simulink model "plant"  (R2022a)
settings: Solver=FixedStepAuto  StartTime=0.0  StopTime=Inf  FixedStep=Ts  RelTol=1e-3  EnableMultiTasking=on
undefined symbols (not defined in the file): A, Analog_max, Calib_Gain, Cd, Crr, D, DiscIntNeverNeededParam, eff_gear, g, Ipeak, Ke, Kf, Kt, La, m_total, n_gear, Offset, Ra, rho, Rwheel, Ts, V_AImax, Vbat, w_motor_max
libraries: c2837xDlib x4, c280xlib x2, simulink x1, c2802xlib x1
settings Model: ExtModeTrigDuration=8  Creator=34688  LastModifiedBy=manu.sanchez
settings SolverCC: AutoInsertRateTranBlk=on
settings OptimizationCC: DefaultUnderspecifiedDataType=single  EnhancedBackFolding=on  PassReuseOutputArgsAs=Individual arguments  MaxStackSize=1024  OptimizeBlockOrder=speed  DifferentSizesBufferReuse=on  OptimizationCustomize=off  DenormalBehavior=FlushToZero  EfficientTunableParamExpr=on
settings DebuggingCC: ParameterTunabilityLossMsg=error  UnconnectedInputMsg=warning  UnconnectedOutputMsg=warning  UnconnectedLineMsg=warning
settings HardwareCC: ProdBitPerChar=16  ProdBitPerInt=16  ProdBitPerPointer=32  ProdBitPerSizeT=32  ProdBitPerPtrDiffT=32  ProdLargestAtomicInteger=Integer  ProdLargestAtomicFloat=None  ProdWordSize=16  ProdLongLongMode=on  ProdHWDeviceType=Texas Instruments->C2000
settings SFSimCC: MATLABDynamicMemAlloc=off
settings RTWCC: SystemTargetFile=ert.tlc  HardwareBoard=TI Delfino F28379D LaunchPad  TemplateMakefile=ert_default_tmf  Toolchain=Texas Instruments Code Composer Studio (C2000)  DLArmComputeVersion=19.05
settings CodeAppCC: ForceParamTrailComments=on  IgnoreCustomStorageClasses=off  OperatorAnnotations=on  SimulinkDataObjDesc=on  SFDataObjDesc=on  InsertBlockDesc=on
settings ERTTargetCC: CodeReplacementLibrary=TI C28x  SupportContinuousTime=on  ExtModeTransport=3  ExtModeStaticAllocSize=10000

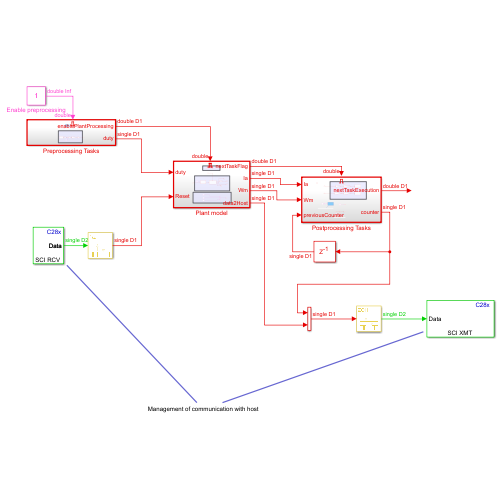
[thumbnail: Simulink's stored preview of the top-level diagram]
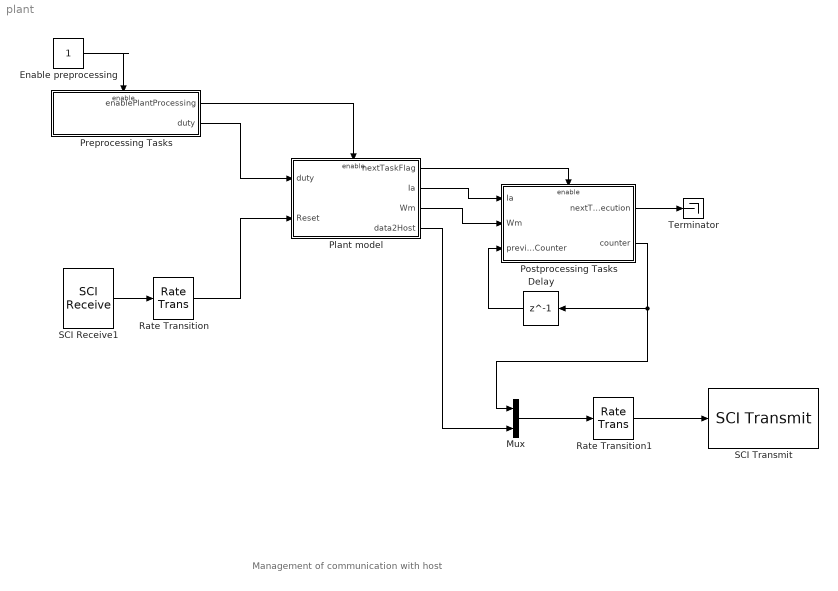
== system plant ==
  note: Management of communication with host
  Delay : Delay  DelayLength=1
  Enable preprocessing : Constant
  Mux : Mux  Inputs=2
  Plant model : Subsystem  TreatAsAtomicUnit=on
  Postprocessing Tasks : Subsystem  TreatAsAtomicUnit=on
  Preprocessing Tasks : Subsystem  TreatAsAtomicUnit=on
  Rate Transition : RateTransition  OutPortSampleTime=Ts
  Rate Transition1 : RateTransition  OutPortSampleTime=1e-3
  SCI Receive1 : c280xlib/SCI Receive  sciModule=A  dataHead='S'  headerCheckMaxCount=16  dataTail='E'  dataType=single  dataLenOptions=Length via dialog  dataDim=1  maxDataLength=1  initValue=0  errOption=Output the last received value  errValue=0  sampleTime=0.001  blockingMode=on  timeOut=0.00875  outputStatus=off
      settings: SourceProductBaseCode=TIC2000
  SCI Transmit : c280xlib/SCI Transmit  sciModule=A  dataHead='S'  dataTail='E'  blockingMode=on  outputStatus=off
  Terminator : Terminator
  wires:
  Plant model/1(nextTaskFlag) -> Postprocessing Tasks/Enable
  Plant model/2(Ia) -> Postprocessing Tasks/1(Ia)
  Enable preprocessing/1 -> Preprocessing Tasks/Enable
  Preprocessing Tasks/1(enablePlantProcessing) -> Plant model/Enable
  Rate Transition/1 -> Plant model/2(Reset)
  SCI Receive1/1 -> Rate Transition/1
  Rate Transition1/1 -> SCI Transmit/1
  Postprocessing Tasks/1(nextTaskExecution) -> Terminator/1
  Delay/1 -> Postprocessing Tasks/3(previousCounter)
  Postprocessing Tasks/2(counter) -> Mux/1, Delay/1
  Mux/1 -> Rate Transition1/1
  Plant model/4(data2Host) -> Mux/2
  Preprocessing Tasks/2(duty) -> Plant model/1(duty)
  Plant model/3(Wm) -> Postprocessing Tasks/2(Wm)

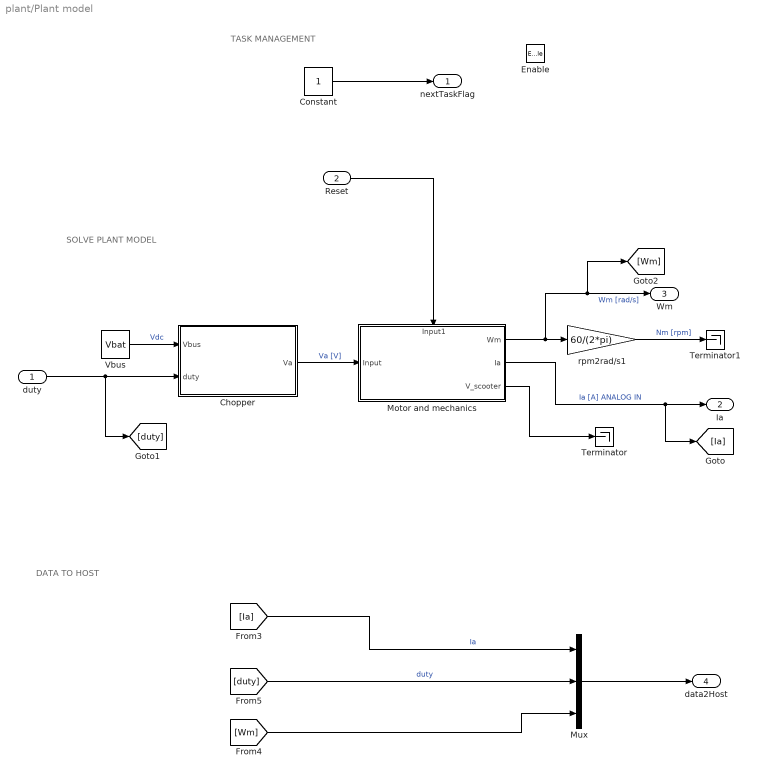
== system plant/Plant model ==
  note: TASK MANAGEMENT
  note: SOLVE PLANT MODEL
  note: DATA TO HOST
  duty : Inport
  Reset : Inport  Port=2
  Enable : EnablePort
  Chopper : Subsystem  Variant=on  VariantControlMode=label  LabelModeActiveChoice=HALF_BRIDGE  mask{LabelModeActiveChoice=HALF_BRIDGE}
      mask prompts: LabelModeActiveChoice "Simulink:Variants:LabelComboBox"
      mask TypeOptions LabelModeActiveChoice: LabelModeActiveChoice
      mask DialogControl LabelModeActiveChoice Prompt: Label mode active choice:
  Constant : Constant  SampleTime=200e-6
  Motor and mechanics : Subsystem
      settings: PortSchema="{\"entries\":[{\"content\":{\"sides\":[{\"content\":{\"connectorIds\":[\"In1\"]},\"type\":\"ConnectorPlacement.EquallySpacedRectSide\",\"uuid\":\"91203ba7-e723-46f9-8594-29464252cc81\"},{\"content\":{\"connectorIds\":[\"Out1\",\"Out2\",\"Out3\"],\"side\":\"RIGHT\"},\"type\":\"ConnectorPlacement.EquallySpacedRectSide\",\"uuid\":\"1e5c0980-dfe5-4f81-9256-2a04590c2b7c\"},{\"content\":{\"connectorIds\":[\"In2\"],\"side\":\"TOP\"},\"type\":\"ConnectorPlacement.EquallySpacedRectSide\",\"uuid\":\"083f4ec4-2b1b-4f60-b44c-9fb8f189a19d\"}]},\"type\":\"ConnectorPlacement.EquallySpacedConnector\",\"uuid\":\"40bc29b3-74aa-4813-97b7-a2598cf603ce\"}],\"packageUris\":[\"http://schema.mathworks.com/mf0/Connector/R2020b\"],\"version\":\"1.0\"}"
  Mux : Mux  Inputs=3
  Terminator : Terminator
  Terminator1 : Terminator
  Vbus : Constant  Value=Vbat  OutDataTypeStr=single
  rpm2rad/s1 : Gain  Gain=60/(2*pi)
  nextTaskFlag : Outport
  Ia : Outport  Port=2
  Wm : Outport  Port=3
  data2Host : Outport  Port=4
  wires:
  Constant/1 -> nextTaskFlag/1
  Motor and mechanics/1(Wm) -> [Wm], Wm/1, rpm2rad/s1/1  "Wm [rad/s]"
  Vbus/1 -> Chopper/1(Vbus)  "Vdc"
  Chopper/1(Va) -> Motor and mechanics/1(Input)  "Va [V]"
  [duty] -> Mux/2  "duty"
  duty/1 -> [duty], Chopper/2(duty)
  [Ia] -> Mux/1  "Ia"
  Motor and mechanics/2(Ia) -> [Ia], Ia/1  "Ia [A] ANALOG IN"
  rpm2rad/s1/1 -> Terminator1/1  "Nm [rpm]"
  Reset/1 -> Motor and mechanics/2(Input1)
  Mux/1 -> data2Host/1
  Motor and mechanics/3(V_scooter) -> Terminator/1
  [Wm] -> Mux/3

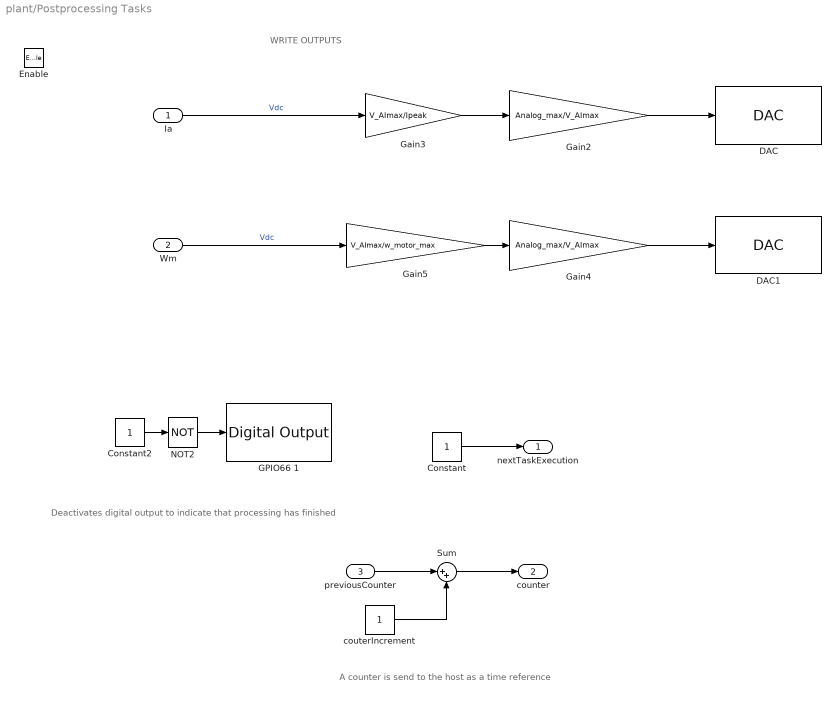
== system plant/Postprocessing Tasks ==
  note: Deactivates digital output to indicate that processing has finished
  note: A counter is send to the host as a time reference
  note: WRITE OUTPUTS
  Ia : Inport
  Wm : Inport  Port=2
  previousCounter : Inport  Port=3
  Enable : EnablePort
  Constant : Constant
  Constant2 : Constant
  DAC : c2837xDlib/DAC  channel=A  saturate=on
      settings: SourceProductBaseCode=TIC2000
  DAC1 : c2837xDlib/DAC  channel=B  saturate=on
      settings: SourceProductBaseCode=TIC2000
  GPIO66 1 : c2837xDlib/Digital Output  GPIO_Number=GPIO0~GPIO7  GPIO_Bit0=on  GPIO_BIT0_Toggle=off  GPIO_Bit1=off  GPIO_BIT1_Toggle=off  GPIO_Bit2=off  GPIO_BIT2_Toggle=off  GPIO_Bit3=off  GPIO_BIT3_Toggle=off  GPIO_Bit4=off  GPIO_BIT4_Toggle=on  GPIO_Bit5=off  GPIO_BIT5_Toggle=on  GPIO_Bit6=off  GPIO_BIT6_Toggle=off  GPIO_Bit7=off  GPIO_BIT7_Toggle=off
      settings: SourceProductBaseCode=TIC2000
  Gain2 : Gain  Gain=Analog_max/V_AImax
  Gain3 : Gain  Gain=V_AImax/Ipeak
  Gain4 : Gain  Gain=Analog_max/V_AImax
  Gain5 : Gain  Gain=V_AImax/w_motor_max
  NOT2 : Logic  Operator=NOT  IconShape=distinctive  AllPortsSameDT=off  OutDataTypeStr=boolean
  Sum : Sum  Inputs=|++
  couterIncrement : Constant  OutDataTypeStr=single
  nextTaskExecution : Outport
  counter : Outport  Port=2
  wires:
  Constant/1 -> nextTaskExecution/1
  Constant2/1 -> NOT2/1
  NOT2/1 -> GPIO66 1/1
  couterIncrement/1 -> Sum/2
  previousCounter/1 -> Sum/1
  Sum/1 -> counter/1
  Gain4/1 -> DAC1/1
  Gain5/1 -> Gain4/1
  Wm/1 -> Gain5/1  "Vdc"
  Gain2/1 -> DAC/1
  Gain3/1 -> Gain2/1
  Ia/1 -> Gain3/1  "Vdc"

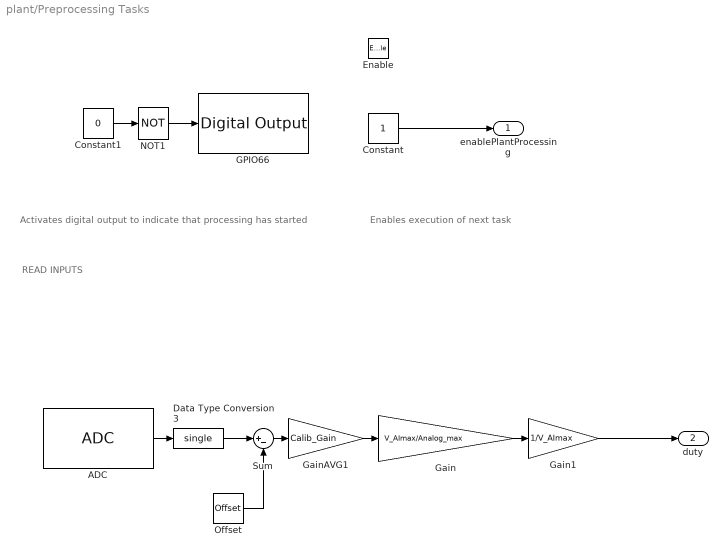
== system plant/Preprocessing Tasks ==
  note: Activates digital output to indicate that processing has started
  note: Enables execution of next task
  note: READ INPUTS
  Enable : EnablePort
  ADC : c2802xlib/ADC  blkParamProc=C2000_Type4  ADCModule=A  samplingMode=Single sample mode  ADCResolution=12-bit (Single-ended input)  useSOC1=SOC0  useSOC2=SOC0_SOC1  SOCAcquisitionWindow=15  SOCTriggerSource=Software  SOCInterruptTrigger=No ADCINT  Ts=Ts  dType=uint16  postInterrupt=off  interruptSel=ADCINT1  ADCINTContinuous=on  endma=off  chdma=1  conv1=ADCINA0  conv2=ADCINA0 and ADCINB0  conv1_Type4=ADCIN15  conv2_Type4=ADCIN0 and ADCIN1
  Constant : Constant
  Constant1 : Constant  Value=0
  Data Type Conversion3 : DataTypeConversion  OutDataTypeStr=single  SaturateOnIntegerOverflow=off  RndMeth=Floor
  "GPIO66 " : c2837xDlib/Digital Output  GPIO_Number=GPIO0~GPIO7  GPIO_Bit0=on  GPIO_BIT0_Toggle=off  GPIO_Bit1=off  GPIO_BIT1_Toggle=off  GPIO_Bit2=off  GPIO_BIT2_Toggle=off  GPIO_Bit3=off  GPIO_BIT3_Toggle=off  GPIO_Bit4=off  GPIO_BIT4_Toggle=on  GPIO_Bit5=off  GPIO_BIT5_Toggle=on  GPIO_Bit6=off  GPIO_BIT6_Toggle=off  GPIO_Bit7=off  GPIO_BIT7_Toggle=off
      settings: SourceProductBaseCode=TIC2000
  Gain : Gain  Gain=V_AImax/Analog_max
  Gain1 : Gain  Gain=1/V_AImax
  GainAVG1 : Gain  Gain=Calib_Gain  OutDataTypeStr=single
  NOT1 : Logic  Operator=NOT  IconShape=distinctive  AllPortsSameDT=off  OutDataTypeStr=boolean
  Offset : Constant  Value=Offset  OutDataTypeStr=single
  Sum : Sum  Inputs=|+-
  enablePlantProcessing : Outport
  duty : Outport  Port=2
  wires:
  Constant/1 -> enablePlantProcessing/1
  Constant1/1 -> NOT1/1
  NOT1/1 -> "GPIO66 "/1
  Gain1/1 -> duty/1
  Gain/1 -> Gain1/1
  GainAVG1/1 -> Gain/1
  ADC/1 -> Data Type Conversion3/1
  Sum/1 -> GainAVG1/1
  Offset/1 -> Sum/2
  Data Type Conversion3/1 -> Sum/1

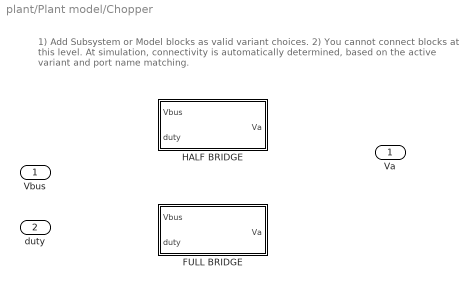
== system plant/Plant model/Chopper ==
  note: 1) Add Subsystem or Model blocks as valid variant choices.
      | 2) You cannot connect blocks at this level. At simulation, connectivity is automatically
      | determined, based on the active variant and port name matching.
  Vbus : Inport
  duty : Inport  Port=2
  FULL BRIDGE : Subsystem  VariantControl=FULL_BRIDGE
  HALF BRIDGE : Subsystem  VariantControl=HALF_BRIDGE
  Va : Outport

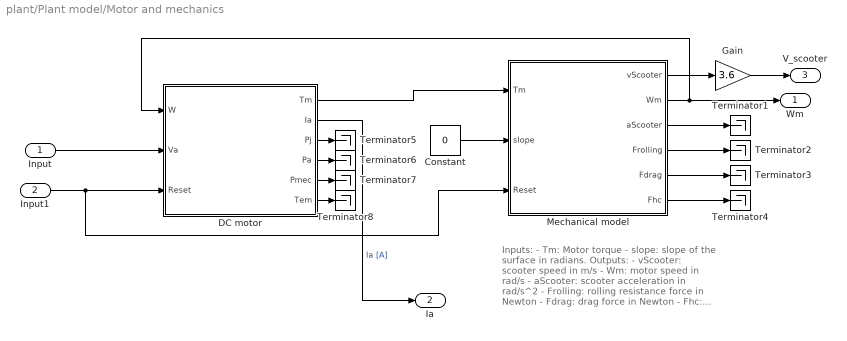
== system plant/Plant model/Motor and mechanics ==
  note: Inputs:
      | - Tm: Motor torque
      | - slope: slope of the surface in radians.
      |
      | Outputs:
      | - vScooter: scooter speed in m/s
      | - Wm: motor speed in rad/s
      | - aScooter: scooter acceleration in rad/s^2
      | - Frolling: rolling resistance force in Newton
      | - Fdrag: drag force in Newton
      | - Fhc: hill climbing force in Newton
  Input : Inport
  Input1 : Inport  Port=2
  Constant : Constant  Value=0  OutDataTypeStr=single
  DC motor : Subsystem
  Gain : Gain  Gain=3.6
  Mechanical model : Subsystem
  Terminator{1..8} (8 alike) : Terminator
  Wm : Outport  VectorParamsAs1DForOutWhenUnconnected=off
  Ia : Outport  Port=2  VectorParamsAs1DForOutWhenUnconnected=off
  V_scooter : Outport  Port=3  VectorParamsAs1DForOutWhenUnconnected=off
  wires:
  Mechanical model/2(Wm) -> Wm/1, DC motor/1(W)
  Input/1 -> DC motor/2(Va)
  Input1/1 -> Mechanical model/3(Reset), DC motor/3(Reset)
  DC motor/2(Ia) -> Ia/1  "Ia [A]"
  Constant/1 -> Mechanical model/2(slope)
  Mechanical model/1(vScooter) -> Gain/1
  Mechanical model/3(aScooter) -> Terminator1/1
  Mechanical model/4(Frolling) -> Terminator2/1
  Mechanical model/5(Fdrag) -> Terminator3/1
  Mechanical model/6(Fhc) -> Terminator4/1
  DC motor/3(Pj) -> Terminator5/1
  DC motor/4(Pa) -> Terminator6/1
  DC motor/5(Pmec) -> Terminator7/1
  DC motor/6(Tem) -> Terminator8/1
  Gain/1 -> V_scooter/1
  DC motor/1(Tm) -> Mechanical model/1(Tm)

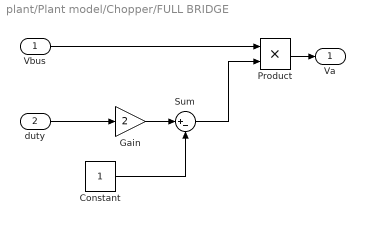
== system plant/Plant model/Chopper/FULL BRIDGE ==
  Vbus : Inport
  duty : Inport  Port=2
  Constant : Constant
  Gain : Gain  Gain=2
  Product : Product
  Sum : Sum  Inputs=|+-
  Va : Outport
  wires:
  duty/1 -> Gain/1
  Gain/1 -> Sum/1
  Constant/1 -> Sum/2
  Product/1 -> Va/1
  Sum/1 -> Product/2
  Vbus/1 -> Product/1

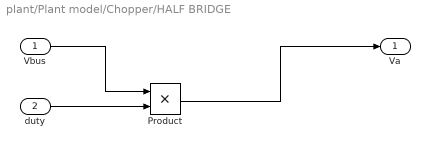
== system plant/Plant model/Chopper/HALF BRIDGE ==
  Vbus : Inport
  duty : Inport  Port=2
  Product : Product
  Va : Outport
  wires:
  Vbus/1 -> Product/1
  duty/1 -> Product/2
  Product/1 -> Va/1

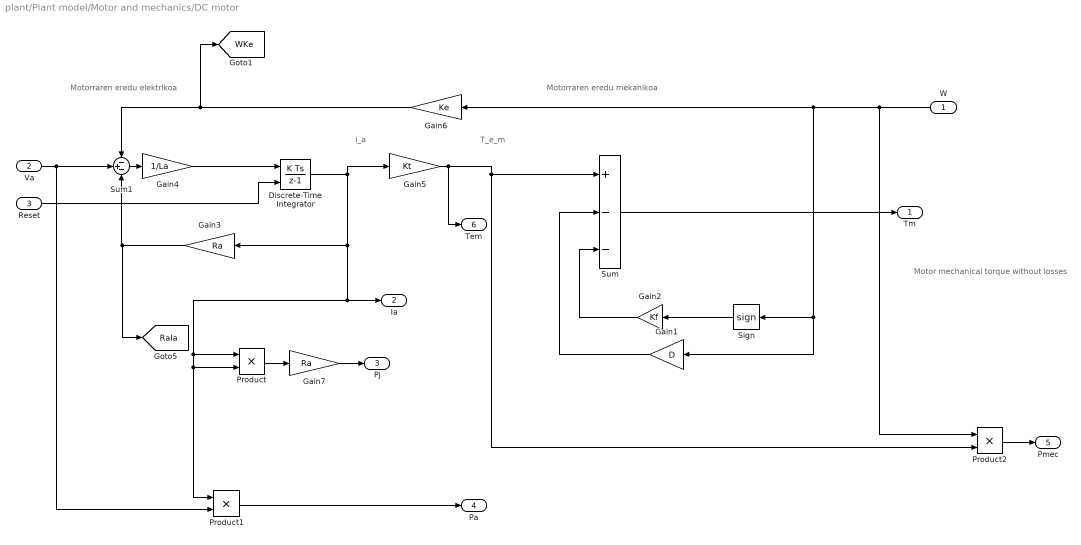
== system plant/Plant model/Motor and mechanics/DC motor ==
  note: Motor mechanical torque without losses
  note: Motorraren eredu mekanikoa
  note: T_e_m
  note: Motorraren eredu elektrikoa
  note: i_a
  W : Inport
  Va : Inport  Port=2
  Reset : Inport  Port=3
  Discrete-Time Integrator : DiscreteIntegrator  ExternalReset=rising  SampleTime=Ts  ICPrevOutput=DiscIntNeverNeededParam  ICPrevScaledInput=DiscIntNeverNeededParam
  Gain1 : Gain  Gain=D
  Gain2 : Gain  Gain=Kf
  Gain3 : Gain  Gain=Ra
  Gain4 : Gain  Gain=1/La
  Gain5 : Gain  Gain=Kt
  Gain6 : Gain  Gain=Ke
  Gain7 : Gain  Gain=Ra
  Product : Product
  Product1 : Product
  Product2 : Product
  Sign : Signum
  Sum : Sum  Inputs=+--
  Sum1 : Sum  Inputs=-+-  AccumDataTypeStr=single
  Tm : Outport  VectorParamsAs1DForOutWhenUnconnected=off
  Ia : Outport  Port=2  VectorParamsAs1DForOutWhenUnconnected=off
  Pj : Outport  Port=3  VectorParamsAs1DForOutWhenUnconnected=off
  Pa : Outport  Port=4  VectorParamsAs1DForOutWhenUnconnected=off
  Pmec : Outport  Port=5  VectorParamsAs1DForOutWhenUnconnected=off
  Tem : Outport  Port=6  VectorParamsAs1DForOutWhenUnconnected=off
  tag scope: RaIa=global, WKe=global
  wires:
  Sum1/1 -> Gain4/1
  Sign/1 -> Gain2/1
  Gain3/1 -> [RaIa], Sum1/3
  Gain1/1 -> Sum/2
  Va/1 -> Product1/2, Sum1/2
  Gain5/1 -> Tem/1, Sum/1, Product2/2
  Sum/1 -> Tm/1
  Discrete-Time Integrator/1 -> Gain5/1, Product/1, Product/2, Product1/1, Ia/1, Gain3/1
  Gain7/1 -> Pj/1
  Product/1 -> Gain7/1
  Product1/1 -> Pa/1
  Product2/1 -> Pmec/1
  Gain2/1 -> Sum/3
  Reset/1 -> Discrete-Time Integrator/2
  W/1 -> Product2/1, Gain1/1, Sign/1, Gain6/1
  Gain6/1 -> [WKe], Sum1/1
  Gain4/1 -> Discrete-Time Integrator/1

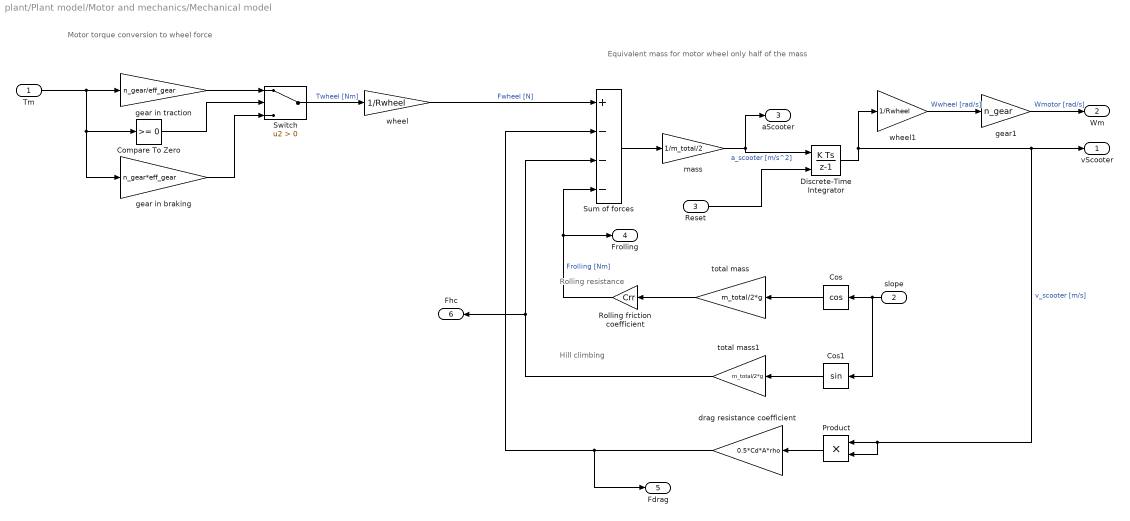
== system plant/Plant model/Motor and mechanics/Mechanical model ==
  note: Hill climbing
  note: Motor torque conversion to wheel force
  note: Equivalent mass for motor wheel only half of the mass
  note: Rolling resistance
  Tm : Inport
  slope : Inport  Port=2
  Reset : Inport  Port=3
  Compare To Zero : simulink/Logic and Bit Operations/Compare To Zero  relop=>=  OutDataTypeStr=boolean
  Cos : Trigonometry  Operator=cos
  Cos1 : Trigonometry
  Discrete-Time Integrator : DiscreteIntegrator  ExternalReset=rising  SampleTime=Ts  ICPrevOutput=DiscIntNeverNeededParam  ICPrevScaledInput=DiscIntNeverNeededParam
  Product : Product
  Rolling friction coefficient : Gain  Gain=Crr
  Sum of forces : Sum  Inputs=+---
  Switch : Switch  Criteria=u2 > Threshold  SaturateOnIntegerOverflow=off  InputSameDT=off
  drag resistance coefficient : Gain  Gain=0.5*Cd*A*rho
  gear in braking : Gain  Gain=n_gear*eff_gear
  gear in traction : Gain  Gain=n_gear/eff_gear
  gear1 : Gain  Gain=n_gear
  mass : Gain  Gain=1/m_total/2
  total mass : Gain  Gain=m_total/2*g
  total mass1 : Gain  Gain=m_total/2*g
  wheel : Gain  Gain=1/Rwheel
  wheel1 : Gain  Gain=1/Rwheel
  vScooter : Outport
  Wm : Outport  Port=2
  aScooter : Outport  Port=3
  Frolling : Outport  Port=4
  Fdrag : Outport  Port=5
  Fhc : Outport  Port=6
  wires:
  Tm/1 -> Compare To Zero/1, gear in braking/1, gear in traction/1
  wheel/1 -> Sum of forces/1  "Fwheel [N]"
  Sum of forces/1 -> mass/1
  mass/1 -> Discrete-Time Integrator/1, aScooter/1  "a_scooter [m/s^2]"
  Discrete-Time Integrator/1 -> Product/2, Product/1, vScooter/1, wheel1/1  "v_scooter [m/s]"
  wheel1/1 -> gear1/1  "Wwheel [rad/s]"
  gear1/1 -> Wm/1  "Wmotor [rad/s]"
  Switch/1 -> wheel/1  "Twheel [Nm]"
  gear in traction/1 -> Switch/1
  gear in braking/1 -> Switch/3
  Compare To Zero/1 -> Switch/2
  Rolling friction coefficient/1 -> Frolling/1, Sum of forces/4  "Frolling [Nm]"
  total mass/1 -> Rolling friction coefficient/1
  Cos/1 -> total mass/1
  slope/1 -> Cos1/1, Cos/1
  Cos1/1 -> total mass1/1
  total mass1/1 -> Fhc/1, Sum of forces/3
  Product/1 -> drag resistance coefficient/1
  drag resistance coefficient/1 -> Fdrag/1, Sum of forces/2
  Reset/1 -> Discrete-Time Integrator/2
